simulink model "sim_quadrotor"  (R2015a)
settings: Solver=ode3  StartTime=0  StopTime=40  FixedStep=sampleTime_qcsim  MaxStep=0.1  RelTol=1e-3
InitFcn:
  | % load parameters of the default quadrotor
  | disp('Quadrotor parameters loaded by InitFcn')
  | paramsFilters %load mdl_quadcopter as well!
  | 
  | % change to Simulation folder if in data folder
  | cd([matlabpath '/Simulation']);
values from neighbouring files (symbols this model uses):
  K_lqr_toMotorcmd = lqr(A,B,Q,R)    [LQRControl.m]
undefined symbols (not defined in the file or in its folder): altEstim, controlParams, Discrete, K_poleplace, ofhandle, quad, quadEDT, sampleTime_qcsim, Time, vishandle
libraries: simulink x29, ctrlSharedLib x3, commnoisgen2 x1
(part 1 of 2)
settings Model: CovSFcnEnable=off  Creator=corkep  LastModifiedBy=root
settings DataIOCC: LimitDataPoints=off  SaveFormat=StructureWithTime  SignalLoggingSaveFormat=ModelDataLogs  SignalLogging=off  DSMLogging=off
settings OptimizationCC: ExpressionDepthLimit=2147483647  OptimizeModelRefInitCode=on  LifeSpan=1
settings DebuggingCC: UnderspecifiedInitializationDetection=Classic  MergeDetectMultiDrivingBlocksExec=none  SolverPrmCheckMsg=warning  FcnCallInpInsideContextMsg=UseLocalSettings  StateNameClashWarn=warning
settings HardwareCC: TargetBitPerLong=64  TargetBitPerPointer=64  TargetLongLongMode=on  TargetIntDivRoundTo=Zero  TargetEndianess=LittleEndian  TargetWordSize=64  TargetHWDeviceType=MATLAB Host  ProdEqTarget=off
settings RTWCC: SystemTargetFile=ert_shrlib.tlc  GenCodeOnly=on  MakeCommand="make_rtw OPTS=\"-DDEFAULT_BUFFER_SIZE=4600\""  GenerateMakefile=off  TemplateMakefile=ert_default_tmf  Description=Embedded Coder (host-based shared library target)  BuildConfiguration=Faster Runs  RTWCompilerOptimization=on
settings CodeAppCC: IgnoreCustomStorageClasses=off
settings STFCustomTargetCC: ParMdlRefBuildCompliant=on  CompOptLevelCompliant=on  IncludeMdlTerminateFcn=off  CombineOutputUpdateFcns=on  MatFileLogging=on  MultiInstanceERTCode=on  CodeInterfacePackaging=Reusable function  SupportContinuousTime=off  SupportVariableSizeSignals=off  ModelStepFunctionPrototypeControlCompliant=on  SystemTargetFile=ert_shrlib.tlc
settings ERTTargetCC: ParMdlRefBuildCompliant=on  CompOptLevelCompliant=on  IncludeMdlTerminateFcn=off  MatFileLogging=on  MultiInstanceERTCode=on  CodeInterfacePackaging=Reusable function  SupportContinuousTime=off  SupportVariableSizeSignals=off  ModelStepFunctionPrototypeControlCompliant=on  MultiInstanceErrorCode=Warning  ERTCustomFileTemplate=example_file_process.tlc

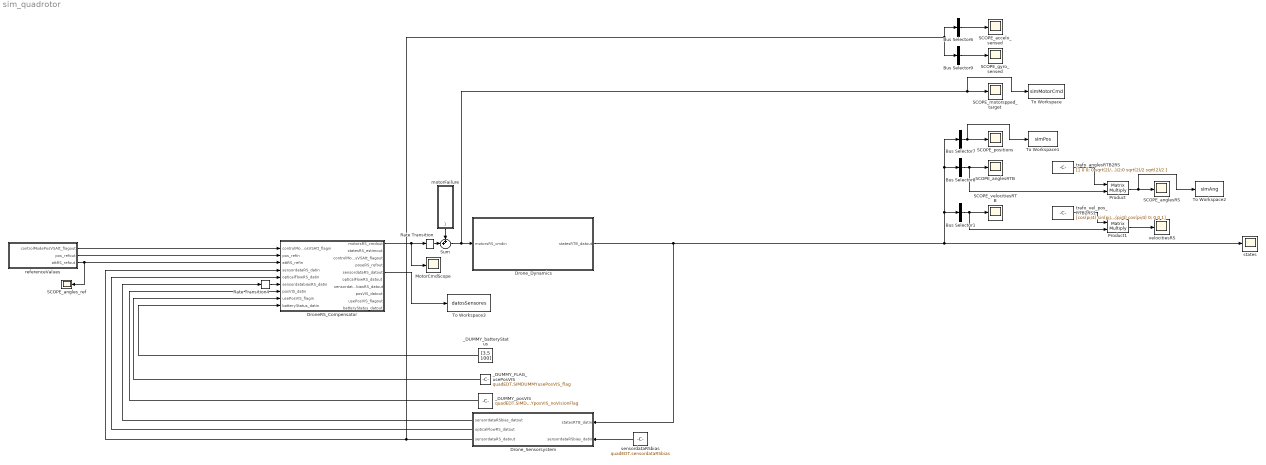
== system sim_quadrotor ==
  Bus Selector1 : BusSelector  OutputSignals=dx,dy,dz  OutputAsBus=on
  Bus Selector6 : BusSelector  OutputSignals=ddx,ddy,ddz  OutputAsBus=on
  Bus Selector7 : BusSelector  OutputSignals=X,Y,Z  OutputAsBus=on
  Bus Selector8 : BusSelector  OutputSignals=yaw,pitch,roll  OutputAsBus=on
  Bus Selector9 : BusSelector  OutputSignals=p,q,r  OutputAsBus=on
  DroneRS_Compensator : Subsystem  TreatAsAtomicUnit=on
  Drone_Dynamics : Subsystem  AncestorBlock=roblocks/Dynamics/Quadrotor
  Drone_Sensorsystem : Subsystem
  "MotorCmdScope " : Scope
      settings: YMin=-300  YMax=300  SaveName=ScopeData6
  Product : Product  Multiplication=Matrix(*)
  Product1 : Product  Multiplication=Matrix(*)
  Rate Transition : RateTransition
  Rate Transition4 : RateTransition  OutPortSampleTime=sampleTime_qcsim
  SCOPE_accelo_sensed : Scope
      settings: TimeRange=14.995  YMin=-13  YMax=2  SaveName=ScopeData11
  SCOPE_anglesRS : Scope
      settings: TimeRange=9.635  YMin=-0.09  YMax=0.06  SaveName=ScopeData8
  SCOPE_anglesRTB : Scope
      settings: TimeRange=10.425  YMin=-0.04  YMax=0.11  SaveName=ScopeData5
  SCOPE_angles_ref : Scope
      settings: TimeRange=15  YMin=-0.15  YMax=0.2  SaveName=ScopeData28
  SCOPE_gyro_sensed : Scope
      settings: TimeRange=14.995  YMin=-0.002  YMax=0.00175  SaveName=ScopeData10
  SCOPE_motorspped_target : Scope
      settings: TimeRange=9.040000000000001  YMin=-400  YMax=400  SaveName=ScopeData2
  SCOPE_positions : Scope
      settings: TimeRange=9.040000000000001  YMin=-0.8  YMax=0.3  SaveName=ScopeData3
  SCOPE_velocitiesRTB : Scope
      settings: TimeRange=13.045  YMin=-1.5  YMax=0.5  SaveName=ScopeData22
  Sum : Sum  Inputs=++|
  To Workspace : ToWorkspace  VariableName=simMotorCmd  SaveFormat=Timeseries  SampleTime=-1
  To Workspace1 : ToWorkspace  VariableName=simPos  SaveFormat=Timeseries  SampleTime=-1
  To Workspace2 : ToWorkspace  VariableName=simAng  SaveFormat=Timeseries  SampleTime=-1
  To Workspace3 : ToWorkspace  VariableName=datosSensores  SaveFormat=Timeseries  SampleTime=-1
  _DUMMY_FLAG_usePosVIS : Constant  Value=quadEDT.SIMDUMMYusePosVIS_flag
  _DUMMY_batteryStatus : Constant  Value=[3.5 100]
  _DUMMY_posVIS : Constant  Value=quadEDT.SIMDUMMYposVIS_noVisionFlag
  motorFailure : Subsystem
  referenceValues : Subsystem
  sensordataRSbias : Constant  Value=quadEDT.sensordataRSbias
  states : Scope
      settings: TimeRange=20  YMin=-1.2  YMax=0.2  SaveName=ScopeData7
  trafo_anglesRTB2RS : Constant  Value=[1 0 0; 0 sqrt(2)/2 -sqrt(2)/2;0 sqrt(2)/2 sqrt(2)/2 ]
  trafo_vel_pos_RTB2RS1 : Constant  Value=[cos(pi/4) sin(pi/4) 0 ; -sin(pi/4) cos(pi/4) 0; 0 0 1]
  velocitiesRS : Scope
      settings: TimeRange=8.18  YMin=-4.991831340204151  YMax=1.573556915322435  SaveName=ScopeData39
  wires:
  Bus Selector7/1 -> To Workspace1/1, SCOPE_positions/1
  Bus Selector8/1 -> Product/2, SCOPE_anglesRTB/1
  Bus Selector6/1 -> SCOPE_accelo_sensed/1
  Bus Selector9/1 -> SCOPE_gyro_sensed/1
  DroneRS_Compensator/1(motorsRS_cmdout) -> "MotorCmdScope "/1, Rate Transition/1
  referenceValues/2("pos_refout ") -> DroneRS_Compensator/2(pos_refin)
  Sum/1 -> To Workspace/1, SCOPE_motorspped_target/1, Drone_Dynamics/1(motorsRS_cmdin)
  motorFailure/1(motorRS_cmdout) -> Sum/1
  Rate Transition/1 -> Sum/2
  referenceValues/1(controlModePosVSAtt_flagout) -> DroneRS_Compensator/1(controlModePosVSAtt_flagin)
  referenceValues/3(attRS_refout) -> DroneRS_Compensator/3(attRS_refin), SCOPE_angles_ref/1
  Drone_Dynamics/1(statesRTB_datout) -> Drone_Sensorsystem/1(statesRTB_datin), states/1, Bus Selector1/1, Bus Selector8/1, Bus Selector7/1
  sensordataRSbias/1 -> Drone_Sensorsystem/2(sensordataRSbias_datin)
  Drone_Sensorsystem/2(opticalFlowRS_datout) -> DroneRS_Compensator/5(opticalFlowRS_datin)
  Rate Transition4/1 -> DroneRS_Compensator/6(sensordatabiasRS_datin)
  Drone_Sensorsystem/3(sensordataRS_datout) -> Bus Selector9/1, Bus Selector6/1, DroneRS_Compensator/4(sensordataRS_datin)
  Drone_Sensorsystem/1(sensordataRSbias_datout) -> Rate Transition4/1
  Product/1 -> To Workspace2/1, SCOPE_anglesRS/1
  trafo_anglesRTB2RS/1 -> Product/1
  _DUMMY_posVIS/1 -> DroneRS_Compensator/7(posVIS_datin)
  Bus Selector1/1 -> Product1/2, SCOPE_velocitiesRTB/1
  Product1/1 -> velocitiesRS/1
  _DUMMY_FLAG_usePosVIS/1 -> DroneRS_Compensator/8(usePosVIS_flagin)
  trafo_vel_pos_RTB2RS1/1 -> Product1/1
  _DUMMY_batteryStatus/1 -> DroneRS_Compensator/9(batteryStatus_datin)
  DroneRS_Compensator/5(sensordataRS_datout) -> To Workspace3/1

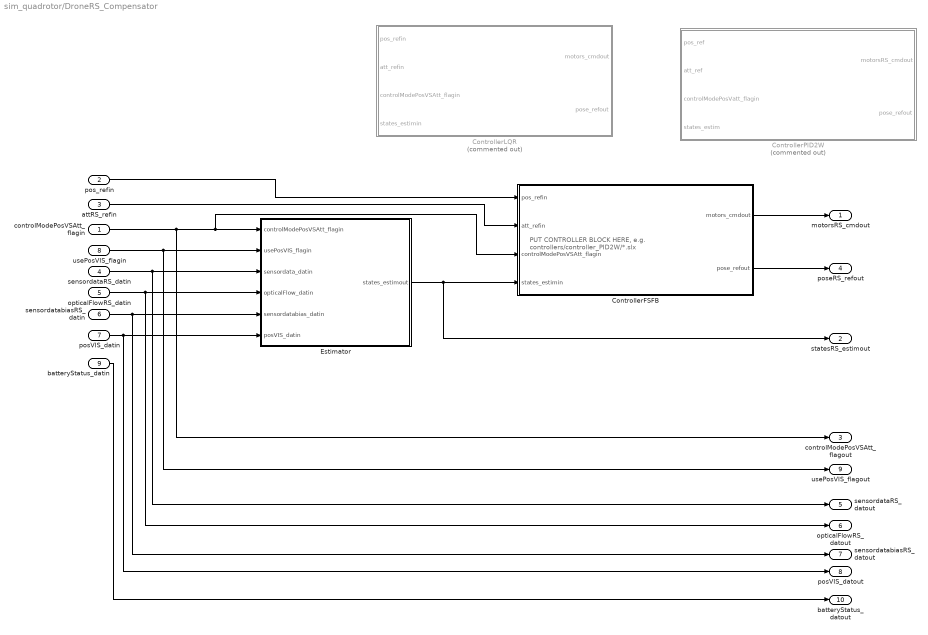
== system sim_quadrotor/DroneRS_Compensator ==
  note: PUT CONTROLLER BLOCK HERE,
      | e.g. controllers/controller_PID2W/*.slx
  controlModePosVSAtt_flagin : Inport
  pos_refin : Inport  Port=2
  attRS_refin : Inport  Port=3
  sensordataRS_datin : Inport  Port=4
  opticalFlowRS_datin : Inport  Port=5
  sensordatabiasRS_datin : Inport  Port=6
  posVIS_datin : Inport  Port=7
  usePosVIS_flagin : Inport  Port=8
  batteryStatus_datin : Inport  Port=9
  ControllerFSFB : Subsystem  TreatAsAtomicUnit=on
  ControllerLQR : Subsystem  Commented=on  TreatAsAtomicUnit=on
  ControllerPID2W : Subsystem  Commented=on  TreatAsAtomicUnit=on
  Estimator : Subsystem
  motorsRS_cmdout : Outport
  statesRS_estimout : Outport  Port=2
  controlModePosVSAtt_flagout : Outport  Port=3
  poseRS_refout : Outport  Port=4
  sensordataRS_datout : Outport  Port=5
  opticalFlowRS_datout : Outport  Port=6
  sensordatabiasRS_datout : Outport  Port=7
  posVIS_datout : Outport  Port=8
  usePosVIS_flagout : Outport  Port=9
  batteryStatus_datout : Outport  Port=10
  wires:
  sensordataRS_datin/1 -> sensordataRS_datout/1, Estimator/3(sensordata_datin)
  pos_refin/1 -> ControllerFSFB/1(pos_refin)
  Estimator/1(states_estimout) -> ControllerFSFB/4(states_estimin), statesRS_estimout/1
  attRS_refin/1 -> ControllerFSFB/2(att_refin)
  controlModePosVSAtt_flagin/1 -> controlModePosVSAtt_flagout/1, ControllerFSFB/3(controlModePosVSAtt_flagin), Estimator/1(controlModePosVSAtt_flagin)
  sensordatabiasRS_datin/1 -> Estimator/5(sensordatabias_datin), sensordatabiasRS_datout/1
  opticalFlowRS_datin/1 -> Estimator/4(opticalFlow_datin), opticalFlowRS_datout/1
  posVIS_datin/1 -> Estimator/6(posVIS_datin), posVIS_datout/1
  usePosVIS_flagin/1 -> usePosVIS_flagout/1, Estimator/2(usePosVIS_flagin)
  batteryStatus_datin/1 -> batteryStatus_datout/1
  ControllerFSFB/1(motors_cmdout) -> motorsRS_cmdout/1
  ControllerFSFB/2(pose_refout) -> poseRS_refout/1

== system sim_quadrotor/Drone_Dynamics ==
  motorsRS_cmdin : Inport
  Bus Creator : BusCreator  Inputs='X','Y','Z','yaw','pitch','roll','dx','dy','dz','p','q','r'
  Demux : Demux  Outputs=12
  Dynamics (Robotics Toolbox Peter Corke) : S-Function  FunctionName=quadrotor_dynamics  Parameters=quad
  MotorsRSToW : Subsystem
  statesRTB_datout : Outport
  wires:
  Demux/1 -> Bus Creator/1  "X"
  Demux/3 -> Bus Creator/3  "Z"
  Demux/4 -> Bus Creator/4  "yaw"
  Demux/5 -> Bus Creator/5  "pitch"
  motorsRS_cmdin/1 -> MotorsRSToW/1(motorsRS_cmdin)
  Demux/7 -> Bus Creator/7  "dx"
  Demux/9 -> Bus Creator/9  "dz"
  Demux/2 -> Bus Creator/2  "Y"
  Demux/6 -> Bus Creator/6  "roll"
  Demux/8 -> Bus Creator/8  "dy"
  Bus Creator/1 -> statesRTB_datout/1
  Dynamics (Robotics Toolbox Peter Corke)/1 -> Demux/1
  Demux/10 -> Bus Creator/10  "p"
  Demux/11 -> Bus Creator/11  "q"
  Demux/12 -> Bus Creator/12  "r"
  MotorsRSToW/1(omega_cmdout) -> Dynamics (Robotics Toolbox Peter Corke)/1

== system sim_quadrotor/Drone_Sensorsystem ==
  statesRTB_datin : Inport
  sensordataRSbias_datin : Inport  Port=2
  IMU_Pressure : Subsystem
  Rate Transition1 : RateTransition  OutPortSampleTime=sampleTime_qcsim
  Rate Transition2 : RateTransition  OutPortSampleTime=sampleTime_qcsim
  camera : Subsystem
  sensordataRSbias_datout : Outport
  opticalFlowRS_datout : Outport  Port=2
  sensordataRS_datout : Outport  Port=3
  wires:
  statesRTB_datin/1 -> IMU_Pressure/2(statesRTB_datin), camera/1(statesRTB_datin)
  sensordataRSbias_datin/1 -> sensordataRSbias_datout/1, IMU_Pressure/1(sensordataRSbias_datin)
  Rate Transition2/1 -> sensordataRS_datout/1
  Rate Transition1/1 -> opticalFlowRS_datout/1
  IMU_Pressure/1(sensordataRS_datout) -> Rate Transition2/1
  camera/1(opticalFlowRS_datout) -> Rate Transition1/1

== system sim_quadrotor/motorFailure ==
  Constant : Constant  Value=0
  Constant1 : Constant  Value=0
  Mux1 : Mux
  Step : Step  Time=quadEDT.motorFailure_time  SampleTime=0
  Step1 : Step  Time=quadEDT.motorFailure_time + quadEDT.motorFailure_duration  SampleTime=0
  Sum : Sum  Inputs=|+-
  motorFailure_gainm2 : Gain  Gain=quadEDT.motorFailure_gainm2
  motorFailure_gainm3 : Gain  Gain=quadEDT.motorFailure_gainm3
  motorRS_cmdout : Outport
  wires:
  Step/1 -> Sum/1
  Step1/1 -> Sum/2
  Sum/1 -> motorFailure_gainm3/1, motorFailure_gainm2/1
  Constant/1 -> Mux1/1
  motorFailure_gainm2/1 -> Mux1/2
  motorFailure_gainm3/1 -> Mux1/3
  Constant1/1 -> Mux1/4
  Mux1/1 -> motorRS_cmdout/1

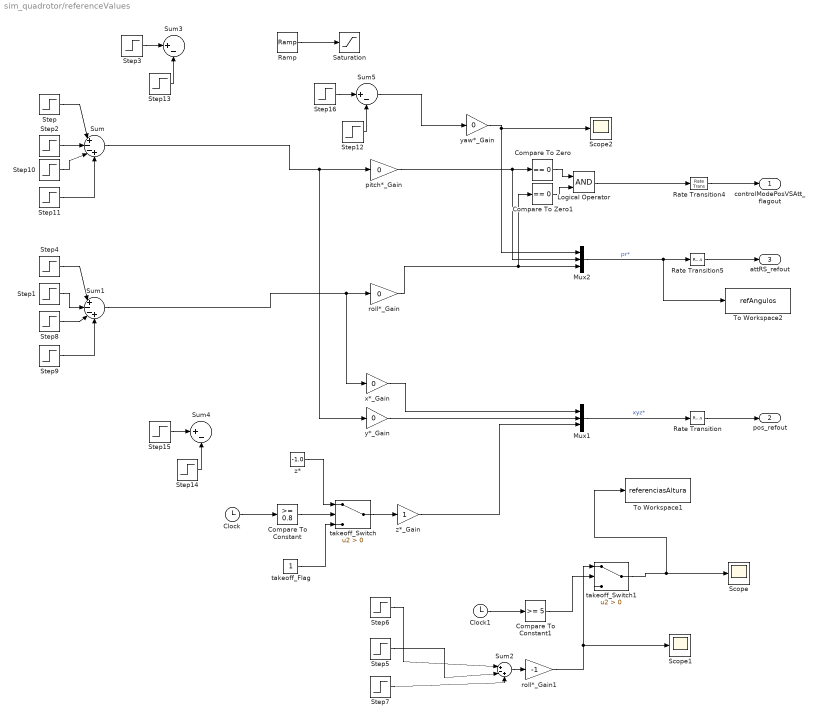
== system sim_quadrotor/referenceValues ==
  Clock : Clock
  Clock1 : Clock
  Compare To Constant : simulink/Logic and Bit Operations/Compare To Constant  relop=>=  const=0.8  OutDataTypeStr=boolean
  Compare To Constant1 : simulink/Logic and Bit Operations/Compare To Constant  relop=>=  const=5  OutDataTypeStr=boolean
  Compare To Zero : simulink/Logic and Bit Operations/Compare To Zero  relop===  OutDataTypeStr=boolean
  Compare To Zero1 : simulink/Logic and Bit Operations/Compare To Zero  relop===  OutDataTypeStr=boolean
  Logical Operator : Logic  AllPortsSameDT=off  OutDataTypeStr=boolean
  Mux1 : Mux  Inputs=3
  Mux2 : Mux  Inputs=3
  Ramp : simulink/Sources/Ramp  slope=1  start=3  X0=0
  Rate Transition : RateTransition  OutPortSampleTime=sampleTime_qcsim
  Rate Transition4 : RateTransition  OutPortSampleTime=sampleTime_qcsim
  Rate Transition5 : RateTransition  OutPortSampleTime=sampleTime_qcsim
  Saturation : Saturate  UpperLimit=5  LowerLimit=-5
  Scope : Scope
      settings: SaveName=ScopeData16
  Scope1 : Scope
      settings: SaveName=ScopeData17
  Scope2 : Scope
      settings: SaveName=ScopeData19
  Step : Step  Time=10  SampleTime=0
  Step1 : Step  Time=8  After=1.001  SampleTime=0
  Step10 : Step  Time=20  SampleTime=0
  Step11 : Step  Time=24  SampleTime=0
  Step12 : Step  Time=18  After=1.001  SampleTime=0
  Step13 : Step  Time=6  After=1.001  SampleTime=0
  Step14 : Step  Time=12  After=1.001  SampleTime=0
  Step15 : Step  Time=9  SampleTime=0
  Step16 : Step  Time=15  SampleTime=0
  Step2 : Step  Time=13  SampleTime=0
  Step3 : Step  Time=3  SampleTime=0
  Step4 : Step  Time=5  SampleTime=0
  Step5 : Step  Time=9  SampleTime=0
  Step6 : Step  Time=5  Before=1  After=1.5  SampleTime=0
  Step7 : Step  Time=12  After=0.5  SampleTime=0
  Step8 : Step  Time=15  SampleTime=0
  Step9 : Step  Time=19  SampleTime=0
  Sum : Sum  Inputs=|+--+
  Sum1 : Sum  Inputs=|+--+
  Sum2 : Sum  Inputs=|+-+
  Sum3 : Sum  Inputs=|+-
  Sum4 : Sum  Inputs=|+-
  Sum5 : Sum  Inputs=|+-
  To Workspace1 : ToWorkspace  VariableName=referenciasAltura  SaveFormat=Timeseries  SampleTime=-1
  To Workspace2 : ToWorkspace  VariableName=refAngulos  SaveFormat=Timeseries  SampleTime=-1
  pitch*_Gain : Gain  Gain=0
  roll*_Gain : Gain  Gain=0
  roll*_Gain1 : Gain  Gain=-1
  takeoff_Flag : Constant  SampleTime=0
  takeoff_Switch : Switch  Criteria=u2 > Threshold
  takeoff_Switch1 : Switch  Criteria=u2 > Threshold
  x*_Gain : Gain  Gain=0
  y*_Gain : Gain  Gain=0
  yaw*_Gain : Gain  Gain=0
  z* : Constant  Value=-1.0  SampleTime=0
  z*_Gain : Gain
  controlModePosVSAtt_flagout : Outport
  "pos_refout " : Outport  Port=2
  attRS_refout : Outport  Port=3
  wires:
  z*/1 -> takeoff_Switch/1
  y*_Gain/1 -> Mux1/2
  Mux1/1 -> Rate Transition/1  "xyz*"
  x*_Gain/1 -> Mux1/1
  Rate Transition/1 -> "pos_refout "/1
  Rate Transition4/1 -> controlModePosVSAtt_flagout/1
  Step/1 -> Sum/1
  Mux2/1 -> To Workspace2/1, Rate Transition5/1  "pr*"
  Rate Transition5/1 -> attRS_refout/1
  Step2/1 -> Sum/2
  yaw*_Gain/1 -> Scope2/1, Mux2/1
  pitch*_Gain/1 -> Mux2/2, Compare To Zero/1
  roll*_Gain/1 -> Mux2/3, Compare To Zero1/1
  Compare To Zero/1 -> Logical Operator/1
  Compare To Zero1/1 -> Logical Operator/2
  Logical Operator/1 -> Rate Transition4/1
  Clock/1 -> Compare To Constant/1
  Compare To Constant/1 -> takeoff_Switch/2
  takeoff_Flag/1 -> takeoff_Switch/3
  takeoff_Switch/1 -> z*_Gain/1
  Clock1/1 -> Compare To Constant1/1
  Compare To Constant1/1 -> takeoff_Switch1/2
  Sum2/1 -> roll*_Gain1/1
  Step6/1 -> Sum2/1
  Step5/1 -> Sum2/2
  roll*_Gain1/1 -> takeoff_Switch1/1, Scope1/1
  takeoff_Switch1/1 -> To Workspace1/1, Scope/1
  Step7/1 -> Sum2/3
  Step10/1 -> Sum/3
  Step11/1 -> Sum/4
  z*_Gain/1 -> Mux1/3
  Sum5/1 -> yaw*_Gain/1
  Step4/1 -> Sum1/1
  Step1/1 -> Sum1/2
  Step8/1 -> Sum1/3
  Step9/1 -> Sum1/4
  Ramp/1 -> Saturation/1
  Step16/1 -> Sum5/1
  Step12/1 -> Sum5/2
  Sum/1 -> y*_Gain/1, pitch*_Gain/1
  Sum1/1 -> x*_Gain/1, roll*_Gain/1
  Step3/1 -> Sum3/1
  Step13/1 -> Sum3/2
  Step15/1 -> Sum4/1
  Step14/1 -> Sum4/2

== system sim_quadrotor/DroneRS_Compensator/ControllerFSFB ==
  pos_refin : Inport
  att_refin : Inport  Port=2
  controlModePosVSAtt_flagin : Inport  Port=3
  states_estimin : Inport  Port=4
  Add : Sum  Inputs=+-
  FullstateController : Subsystem
  Selector : Selector  InputPortWidth=12  Indices=[1:6]
  SysteminputConverter : Subsystem
  statesReferences : Subsystem
  motors_cmdout : Outport
  pose_refout : Outport  Port=2
  wires:
  Selector/1 -> pose_refout/1
  statesReferences/2(states_refout) -> Add/1, Selector/1
  controlModePosVSAtt_flagin/1 -> statesReferences/3(controlModePosVSAtt_flagin)
  states_estimin/1 -> statesReferences/4(states_estimin), Add/2
  att_refin/1 -> statesReferences/2(att_refin)
  pos_refin/1 -> statesReferences/1(pos_refin)
  Add/1 -> FullstateController/1(state_error_datin)  "state error e"
  statesReferences/1(takeoffphase_flagout) -> SysteminputConverter/1(takeoffphase_flagin)
  FullstateController/1(u_totThrust_Torques_refout) -> SysteminputConverter/2(u_totThrust_Torques_refin)
  SysteminputConverter/1(motors_cmdout) -> motors_cmdout/1

== system sim_quadrotor/DroneRS_Compensator/ControllerLQR ==
  pos_refin : Inport
  att_refin : Inport  Port=2
  controlModePosVSAtt_flagin : Inport  Port=3
  states_estimin : Inport  Port=4
  Add : Sum  Inputs=+-
  FullstateController : Subsystem
  Selector : Selector  InputPortWidth=12  Indices=[1:6]
  SysteminputConverter : Subsystem
  statesReferences : Subsystem
  motors_cmdout : Outport
  pose_refout : Outport  Port=2
  wires:
  statesReferences/2(states_refout) -> Add/1, Selector/1
  controlModePosVSAtt_flagin/1 -> statesReferences/3(controlModePosVSAtt_flagin)
  states_estimin/1 -> statesReferences/4(states_estimin), Add/2
  att_refin/1 -> statesReferences/2(att_refin)
  Add/1 -> FullstateController/1(state_error_datin)  "state error e"
  statesReferences/1(takeoffphase_flagout) -> SysteminputConverter/1(takeoffphase_flagin)
  FullstateController/1(motors_cmdout) -> SysteminputConverter/2(motors_cmdin)
  pos_refin/1 -> statesReferences/1(pos_refin)
  SysteminputConverter/1(motors_cmdout) -> motors_cmdout/1
  Selector/1 -> pose_refout/1

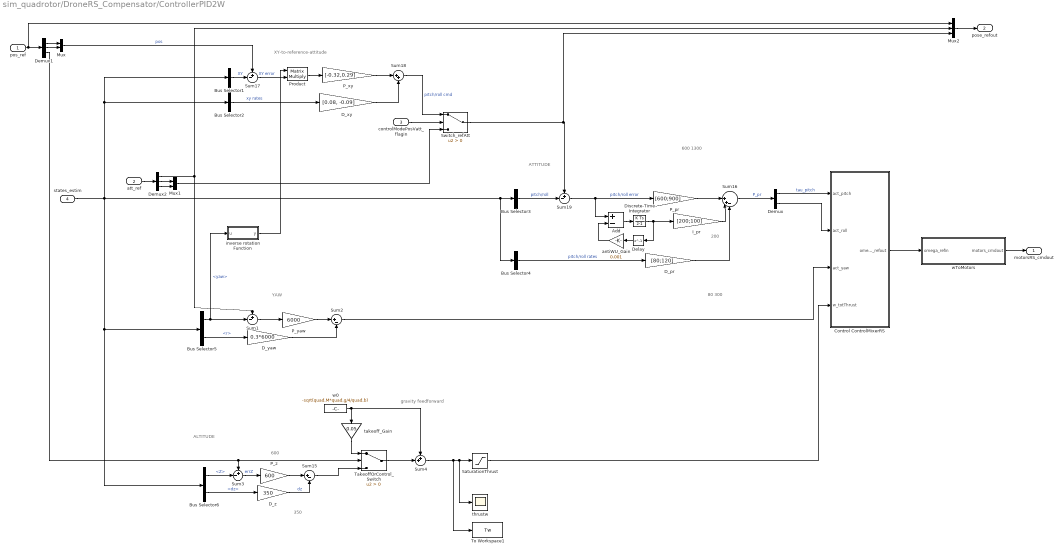
== system sim_quadrotor/DroneRS_Compensator/ControllerPID2W ==
  note: 350
  note: 600
  note: 200
  note: 80 300
  note: 600 1300
  note: XY-to-reference-attitude
  note: ALTITUDE
  note: ATTITUDE
  note: YAW
  note: gravity feedforward
  pos_ref : Inport
  att_ref : Inport  Port=2
  controlModePosVatt_flagin : Inport  Port=3
  states_estim : Inport  Port=4
  Add : Sum  Inputs=+-
  Bus Selector1 : BusSelector  OutputSignals=X,Y  OutputAsBus=on
  Bus Selector2 : BusSelector  OutputSignals=dx,dy  OutputAsBus=on
  Bus Selector3 : BusSelector  OutputSignals=pitch,roll  OutputAsBus=on
  Bus Selector4 : BusSelector  OutputSignals=q,p  OutputAsBus=on
  Bus Selector5 : BusSelector  OutputSignals=yaw,r
  Bus Selector6 : BusSelector  OutputSignals=Z,dz
  Control ControlMixerRS : Subsystem
  D_pr : Gain  Gain=[80;120]
  D_xy : Gain  Gain=[0.08, -0.09]
  D_yaw : Gain  Gain=0.3*6000
  D_z : Gain  Gain=350
  Delay : Delay  DelayLength=1  InitialCondition=0
  Demux : Demux  Outputs=2
  Demux1 : Demux  Outputs=3
  Demux2 : Demux  Outputs=3
  Discrete-Time Integrator : DiscreteIntegrator  InitialConditionSetting=State (most efficient)  SampleTime=sampleTime_qcsim  LimitOutput=on  UpperSaturationLimit=2  LowerSaturationLimit=-2
  I_pr : Gain  Gain=[200;100]
  Mux : Mux  Inputs=2
  Mux1 : Mux  Inputs=2
  Mux2 : Mux  Inputs=3
  P_pr : Gain  Gain=[600;900]
  P_xy : Gain  Gain=[-0.32,0.29]
  P_yaw : Gain  Gain=6000
  P_z : Gain  Gain=600
  Product : Product  Multiplication=Matrix(*)  RndMeth=Zero
  SaturationThrust : Saturate  UpperLimit=0.92*2618  LowerLimit=-0.92*2618
  Sum{1,3,17,19} (4 alike) : Sum  Inputs=+-|
  Sum15 : Sum  Inputs=|+-
  Sum16 : Sum  Inputs=||++-
  Sum18 : Sum  Inputs=|++
  Sum2 : Sum  Inputs=|+-
  Sum4 : Sum  Inputs=++|
  Switch_refAtt : Switch  Criteria=u2 > Threshold
  TakeoffOrControl_Switch : Switch  Criteria=u2 > Threshold
  To Workspace1 : ToWorkspace  VariableName=Tw  SampleTime=-1
  antiWU_Gain : Gain  Gain=0.001
  inverse rotation Function : MATLAB Function  TreatAsAtomicUnit=on
  takeoff_Gain : Gain  Gain=0.05
  thrustw : Scope
      settings: YMin=-0.04  YMax=0.045  SaveName=ScopeData15
  w0 : Constant  Value=-sqrt(quad.M*quad.g/4/quad.b)  SampleTime=sampleTime_qcsim
  wToMotors : Subsystem
  motorsRS_cmdout : Outport
  pose_refout : Outport  Port=2
  wires:
  w0/1 -> takeoff_Gain/1, Sum4/1
  Bus Selector2/1 -> D_xy/1  "xy rates"
  Bus Selector4/1 -> D_pr/1  "pitch/roll rates"
  Sum19/1 -> P_pr/1, Add/1  "pitch/roll error"
  Sum16/1 -> Demux/1  "P_pr"
  Bus Selector5/1 -> inverse rotation Function/1(u), Sum1/2  "<yaw>"
  Bus Selector6/1 -> Sum3/2  "<Z>"
  inverse rotation Function/1(y) -> Product/1
  Bus Selector5/2 -> D_yaw/1  "<r>"
  Sum3/1 -> P_z/1  "errZ"
  Bus Selector6/2 -> D_z/1  "<dz>"
  D_z/1 -> Sum15/2  "dz"
  D_yaw/1 -> Sum2/2
  Sum4/1 -> To Workspace1/1, thrustw/1, SaturationThrust/1
  Sum1/1 -> P_yaw/1
  Sum17/1 -> Product/2  "XY error"
  Discrete-Time Integrator/1 -> Delay/1, I_pr/1
  Demux/1 -> Control ControlMixerRS/1(act_pitch)  "tau_pitch"
  Sum2/1 -> Control ControlMixerRS/3(act_yaw)
  Demux/2 -> Control ControlMixerRS/2(act_roll)
  TakeoffOrControl_Switch/1 -> Sum4/2
  Sum15/1 -> TakeoffOrControl_Switch/3
  takeoff_Gain/1 -> TakeoffOrControl_Switch/1
  Sum18/1 -> Switch_refAtt/1  "pitch/roll cmd"
  controlModePosVatt_flagin/1 -> Switch_refAtt/2
  pos_ref/1 -> Mux2/1, Demux1/1
  Demux1/1 -> Mux/1
  Demux1/2 -> Mux/2
  Mux/1 -> Sum17/1  "pos"
  Demux2/2 -> Mux1/1
  Demux2/3 -> Mux1/2
  att_ref/1 -> Demux2/1
  Mux1/1 -> Switch_refAtt/3
  Demux2/1 -> Mux2/2, Sum1/1
  Demux1/3 -> Sum3/1, TakeoffOrControl_Switch/2
  Bus Selector3/1 -> Sum19/2  "pitch/roll"
  Product/1 -> P_xy/1
  D_xy/1 -> Sum18/2
  Bus Selector1/1 -> Sum17/2  "XY"
  P_z/1 -> Sum15/1
  SaturationThrust/1 -> Control ControlMixerRS/4(w_totThrust)
  P_yaw/1 -> Sum2/1
  I_pr/1 -> Sum16/2
  D_pr/1 -> Sum16/3
  P_pr/1 -> Sum16/1
  Control ControlMixerRS/1(omega_refout) -> wToMotors/1(omega_refin)
  wToMotors/1(motors_cmdout) -> motorsRS_cmdout/1
  Mux2/1 -> pose_refout/1
  Switch_refAtt/1 -> Mux2/3, Sum19/1
  states_estim/1 -> Bus Selector4/1, Bus Selector3/1, Bus Selector1/1, Bus Selector2/1, Bus Selector5/1, Bus Selector6/1
  P_xy/1 -> Sum18/1
  Add/1 -> Discrete-Time Integrator/1
  antiWU_Gain/1 -> Add/2
  Delay/1 -> antiWU_Gain/1

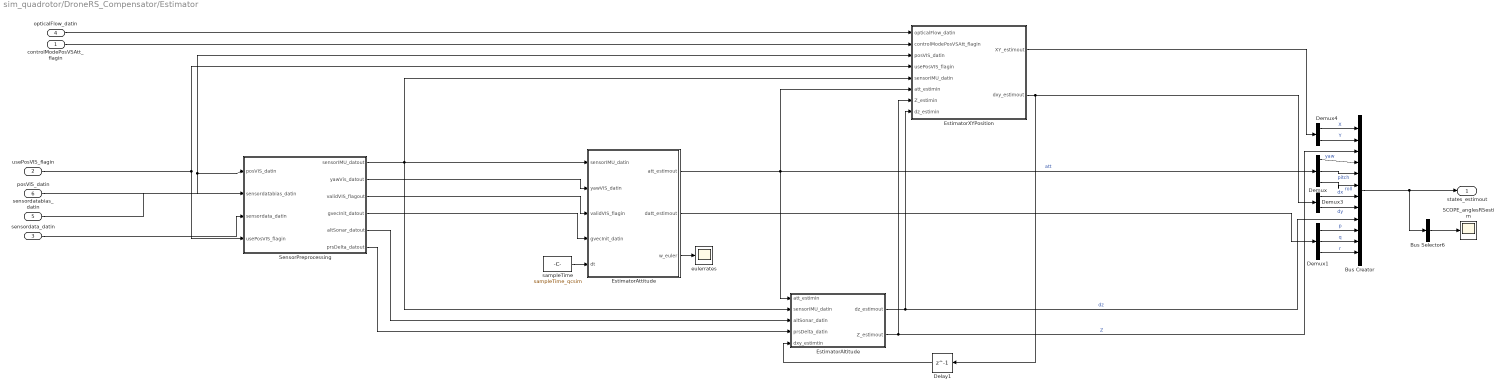
== system sim_quadrotor/DroneRS_Compensator/Estimator ==
  controlModePosVSAtt_flagin : Inport
  usePosVIS_flagin : Inport  Port=2
  sensordata_datin : Inport  Port=3
  opticalFlow_datin : Inport  Port=4
  sensordatabias_datin : Inport  Port=5
  posVIS_datin : Inport  Port=6
  Bus Creator : BusCreator  Inputs='X','Y','Z','yaw','pitch','roll','dx','dy','dz','p','q','r'
  Bus Selector6 : BusSelector  OutputSignals=yaw,pitch,roll  OutputAsBus=on
  Delay1 : Delay  DelayLength=1  InitialCondition=0
  Demux : Demux  Outputs=3
  Demux1 : Demux  Outputs=3
  Demux3 : Demux  Outputs=2
  Demux4 : Demux  Outputs=2
  EstimatorAltitude : Subsystem
  EstimatorAttitude : MATLAB Function  TreatAsAtomicUnit=on
  EstimatorXYPosition : Subsystem
  SCOPE_anglesRSestim : Scope
      settings: TimeRange=3.57  YMin=-0.08  YMax=0.06000000000000001  SaveName=ScopeData4
  SensorPreprocessing : Subsystem
  eulerrates : Scope
      settings: SaveName=ScopeData18
  sampleTime : Constant  Value=sampleTime_qcsim
  states_estimout : Outport
  wires:
  Bus Creator/1 -> Bus Selector6/1, states_estimout/1
  sampleTime/1 -> EstimatorAttitude/5(dt)
  sensordatabias_datin/1 -> SensorPreprocessing/2(sensordatabias_datin)
  EstimatorAttitude/3(w_euler) -> eulerrates/1
  EstimatorAltitude/2(Z_estimout) -> Bus Creator/3, EstimatorXYPosition/7(Z_estimin)  "Z"
  EstimatorAltitude/1(dz_estimout) -> Bus Creator/9, EstimatorXYPosition/8(dz_estimin)  "dz"
  opticalFlow_datin/1 -> EstimatorXYPosition/1(opticalFlow_datin)
  Demux3/1 -> Bus Creator/7  "dx"
  Demux3/2 -> Bus Creator/8  "dy"
  EstimatorXYPosition/2(dxy_estimout) -> Delay1/1, Demux3/1
  Delay1/1 -> EstimatorAltitude/5(dxy_estimtin)
  controlModePosVSAtt_flagin/1 -> EstimatorXYPosition/2(controlModePosVSAtt_flagin)
  Demux4/1 -> Bus Creator/1  "X"
  Demux4/2 -> Bus Creator/2  "Y"
  EstimatorXYPosition/1(XY_estimout) -> Demux4/1
  posVIS_datin/1 -> EstimatorXYPosition/3(posVIS_datin), SensorPreprocessing/1(posVIS_datin)
  usePosVIS_flagin/1 -> SensorPreprocessing/4(usePosVIS_flagin), EstimatorXYPosition/4(usePosVIS_flagin)
  Bus Selector6/1 -> SCOPE_anglesRSestim/1
  SensorPreprocessing/1(sensorIMU_datout) -> EstimatorAltitude/2(sensorIMU_datin), EstimatorXYPosition/5(sensorIMU_datin), EstimatorAttitude/1(sensorIMU_datin)
  SensorPreprocessing/4(gvecInit_datout) -> EstimatorAttitude/4(gvecInit_datin)
  sensordata_datin/1 -> SensorPreprocessing/3(sensordata_datin)
  SensorPreprocessing/5(altSonar_datout) -> EstimatorAltitude/3(altSonar_datin)
  SensorPreprocessing/6(prsDelta_datout) -> EstimatorAltitude/4(prsDelta_datin)
  EstimatorAttitude/1(att_estimout) -> EstimatorAltitude/1(att_estimin), Demux/1, EstimatorXYPosition/6(att_estimin)  "att"
  Demux/1 -> Bus Creator/4  "yaw"
  Demux/2 -> Bus Creator/5  "pitch"
  Demux/3 -> Bus Creator/6  "roll"
  Demux1/1 -> Bus Creator/10  "p"
  Demux1/2 -> Bus Creator/11  "q"
  Demux1/3 -> Bus Creator/12  "r"
  EstimatorAttitude/2(datt_estimout) -> Demux1/1
  SensorPreprocessing/3(validVIS_flagout) -> EstimatorAttitude/3(validVIS_flagin)
  SensorPreprocessing/2(yawVis_datout) -> EstimatorAttitude/2(yawVIS_datin)

== system sim_quadrotor/Drone_Dynamics/MotorsRSToW ==
  motorsRS_cmdin : Inport
  Signed Sqrt : Sqrt  Operator=signedSqrt  SaturateOnIntegerOverflow=on
  motorsRSToW2_Gain : Gain  Gain=quadEDT.motorsRSToW2_Gain
  omega_cmdout : Outport
  wires:
  motorsRSToW2_Gain/1 -> Signed Sqrt/1
  motorsRS_cmdin/1 -> motorsRSToW2_Gain/1
  Signed Sqrt/1 -> omega_cmdout/1

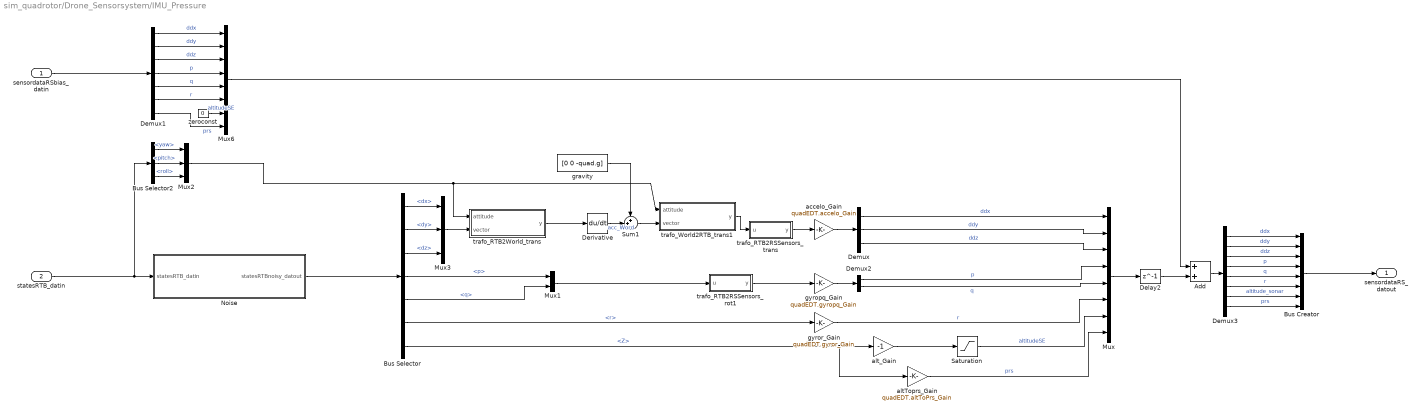
== system sim_quadrotor/Drone_Sensorsystem/IMU_Pressure ==
  sensordataRSbias_datin : Inport
  statesRTB_datin : Inport  Port=2
  " Noise" : Subsystem
  Add : Sum
  Bus Creator : BusCreator  Inputs=8
  Bus Selector : BusSelector  OutputSignals=dx,dy,dz,p,q,r,Z
  Bus Selector2 : BusSelector  OutputSignals=yaw,pitch,roll
  Delay2 : Delay  DelayLength=1  InitialCondition=0
  Demux : Demux  Outputs=3
  Demux1 : Demux  Outputs=7
  Demux2 : Demux  Outputs=2
  Demux3 : Demux  Outputs=8
  Derivative : Derivative
  Mux : Mux  Inputs=8
  Mux1 : Mux  Inputs=2
  Mux2 : Mux  Inputs=3
  Mux3 : Mux  Inputs=3
  Mux6 : Mux  Inputs=8
  Saturation : Saturate  UpperLimit=inf  LowerLimit=quadEDT.altSenor_LowerLimit
  Sum1 : Sum  Inputs=++|
  accelo_Gain : Gain  Gain=quadEDT.accelo_Gain
  altToprs_Gain : Gain  Gain=quadEDT.altToPrs_Gain
  alt_Gain : Gain  Gain=-1
  gravity : Constant  Value=[0 0 -quad.g]
  gyropq_Gain : Gain  Gain=quadEDT.gyropq_Gain
  gyror_Gain : Gain  Gain=quadEDT.gyror_Gain
  trafo_RTB2RSSensors_rot1 : MATLAB Function  TreatAsAtomicUnit=on
  trafo_RTB2RSSensors_trans : MATLAB Function  TreatAsAtomicUnit=on
  trafo_RTB2World_trans : MATLAB Function  TreatAsAtomicUnit=on
  trafo_World2RTB_trans1 : MATLAB Function  TreatAsAtomicUnit=on
  zeroconst : Constant  Value=0
  sensordataRS_datout : Outport
  wires:
  statesRTB_datin/1 -> " Noise"/1(statesRTB_datin), Bus Selector2/1
  sensordataRSbias_datin/1 -> Demux1/1
  Demux2/2 -> Mux/5  "q"
  Demux2/1 -> Mux/4  "p"
  " Noise"/1(statesRTBnoisy_datout) -> Bus Selector/1
  Bus Selector/2 -> Mux3/2  "<dy>"
  trafo_RTB2RSSensors_trans/1(y) -> accelo_Gain/1
  Demux/1 -> Mux/1  "ddx"
  Demux/2 -> Mux/2  "ddy"
  gyror_Gain/1 -> Mux/6  "r"
  Bus Selector2/1 -> Mux2/1  "<yaw>"
  Bus Selector2/2 -> Mux2/2  "<pitch>"
  Bus Selector2/3 -> Mux2/3  "<roll>"
  Demux/3 -> Mux/3  "ddz"
  Mux2/1 -> trafo_World2RTB_trans1/1(attitude), trafo_RTB2World_trans/1(attitude)
  gravity/1 -> Sum1/1
  Mux1/1 -> trafo_RTB2RSSensors_rot1/1(u)
  Bus Selector/4 -> Mux1/1  "<p>"
  Bus Selector/5 -> Mux1/2  "<q>"
  Bus Selector/6 -> gyror_Gain/1  "<r>"
  Bus Selector/7 -> altToprs_Gain/1, alt_Gain/1  "<Z>"
  alt_Gain/1 -> Saturation/1
  Saturation/1 -> Mux/7  "altitudeSE"
  Bus Selector/3 -> Mux3/3  "<dz>"
  altToprs_Gain/1 -> Mux/8  "prs"
  Demux1/1 -> Mux6/1  "ddx"
  Demux1/2 -> Mux6/2  "ddy"
  Demux1/3 -> Mux6/3  "ddz"
  Demux1/4 -> Mux6/4  "p"
  Demux1/5 -> Mux6/5  "q"
  Demux1/6 -> Mux6/6  "r"
  zeroconst/1 -> Mux6/7  "altitudeSE"
  Demux1/7 -> Mux6/8  "prs"
  Mux6/1 -> Add/1
  Add/1 -> Demux3/1
  Mux/1 -> Delay2/1
  Demux3/3 -> Bus Creator/3  "ddz"
  Demux3/1 -> Bus Creator/1  "ddx"
  Demux3/2 -> Bus Creator/2  "ddy"
  Demux3/4 -> Bus Creator/4  "p"
  Demux3/5 -> Bus Creator/5  "q"
  Demux3/6 -> Bus Creator/6  "r"
  Demux3/7 -> Bus Creator/7  "altitude_sonar"
  Demux3/8 -> Bus Creator/8  "prs"
  Bus Creator/1 -> sensordataRS_datout/1
  trafo_RTB2RSSensors_rot1/1(y) -> gyropq_Gain/1
  Bus Selector/1 -> Mux3/1  "<dx>"
  Delay2/1 -> Add/2
  accelo_Gain/1 -> Demux/1
  gyropq_Gain/1 -> Demux2/1
  Mux3/1 -> trafo_RTB2World_trans/2(vector)
  trafo_RTB2World_trans/1(y) -> Derivative/1
  Sum1/1 -> trafo_World2RTB_trans1/2(vector)
  Derivative/1 -> Sum1/2  "acc_Word"
  trafo_World2RTB_trans1/1(y) -> trafo_RTB2RSSensors_trans/1(u)

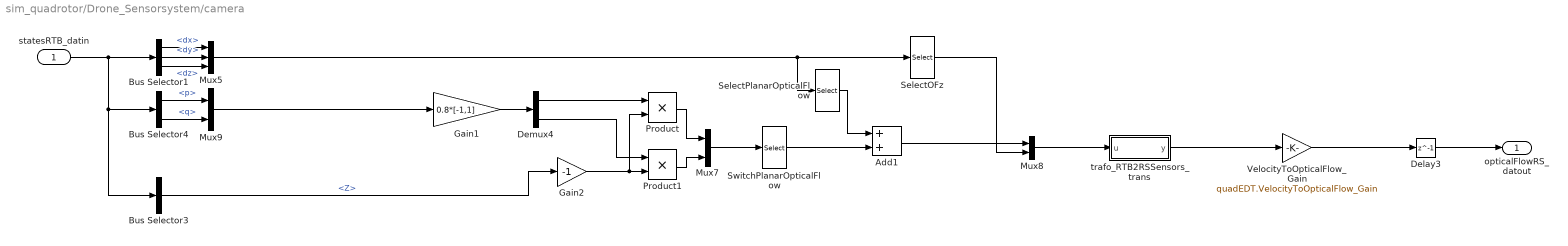
== system sim_quadrotor/Drone_Sensorsystem/camera ==
  statesRTB_datin : Inport
  Add1 : Sum
  Bus Selector1 : BusSelector  OutputSignals=dx,dy,dz
  Bus Selector3 : BusSelector  OutputSignals=Z
  Bus Selector4 : BusSelector  OutputSignals=p,q
  Delay3 : Delay  DelayLength=1  InitialCondition=0
  Demux4 : Demux  Outputs=2
  Gain1 : Gain  Gain=0.8*[-1,1]
  Gain2 : Gain  Gain=-1
  Mux5 : Mux  Inputs=3
  Mux7 : Mux  Inputs=2
  Mux8 : Mux  Inputs=2
  Mux9 : Mux  Inputs=2
  Product : Product
  Product1 : Product
  SelectOFz : Selector  InputPortWidth=3  Indices=3
  SelectPlanarOpticalFlow : Selector  InputPortWidth=3  Indices=[1 2]
  SwitchPlanarOpticalFlow : Selector  InputPortWidth=2  Indices=[2 1]
  VelocityToOpticalFlow_Gain : Gain  Gain=quadEDT.VelocityToOpticalFlow_Gain
  trafo_RTB2RSSensors_trans : MATLAB Function  TreatAsAtomicUnit=on
  opticalFlowRS_datout : Outport
  wires:
  statesRTB_datin/1 -> Bus Selector3/1, Bus Selector4/1, Bus Selector1/1
  Bus Selector1/1 -> Mux5/1  "<dx>"
  Bus Selector1/2 -> Mux5/2  "<dy>"
  Bus Selector1/3 -> Mux5/3  "<dz>"
  VelocityToOpticalFlow_Gain/1 -> Delay3/1
  Mux5/1 -> SelectPlanarOpticalFlow/1, SelectOFz/1
  Demux4/1 -> Product/1
  Gain1/1 -> Demux4/1
  Demux4/2 -> Product1/1
  Product/1 -> Mux7/1
  Product1/1 -> Mux7/2
  Mux7/1 -> SwitchPlanarOpticalFlow/1
  Mux9/1 -> Gain1/1
  Gain2/1 -> Product/2, Product1/2
  SelectPlanarOpticalFlow/1 -> Add1/1
  SwitchPlanarOpticalFlow/1 -> Add1/2
  Add1/1 -> Mux8/1
  SelectOFz/1 -> Mux8/2
  Mux8/1 -> trafo_RTB2RSSensors_trans/1(u)
  Bus Selector3/1 -> Gain2/1  "<Z>"
  Bus Selector4/1 -> Mux9/1  "<p>"
  Bus Selector4/2 -> Mux9/2  "<q>"
  trafo_RTB2RSSensors_trans/1(y) -> VelocityToOpticalFlow_Gain/1
  Delay3/1 -> opticalFlowRS_datout/1

== system sim_quadrotor/DroneRS_Compensator/ControllerFSFB/FullstateController ==
  note: IMPLEMENT FULLSTATE-
      | CONTROLLER HERE
  state_error_datin : Inport
  Gain : Gain  Gain=K_poleplace  Multiplication=Matrix(K*u)
  u_totThrust_Torques_refout : Outport
  wires:
  state_error_datin/1 -> Gain/1
  Gain/1 -> u_totThrust_Torques_refout/1

== system sim_quadrotor/DroneRS_Compensator/ControllerFSFB/SysteminputConverter ==
  note: NOTE: The Systeminputconverter takes care of two things:
      | 1) During take off, adjust the total thrust proposed by the controller
      | 2) Translate the "mechanical" system inputs (total thrust, torques around body-frame x-y-z-axes) to actual motor commands.
      | This R4->R4 mapping is a simple bijective function and does not have any dynamics. This allows us to design the controller with more intuitive "mechanical inputs" (total thrust, torques) and later simple map these to actual motor commands.
  takeoffphase_flagin : Inport
  u_totThrust_Torques_refin : Inport  Port=2
  ControlMixerRS : Subsystem
  Demux3 : Demux
  Takeoffphase_Thrustadjustment : Subsystem
  Thrust2Motorcmd : Subsystem
  motors_cmdout : Outport
  wires:
  takeoffphase_flagin/1 -> Takeoffphase_Thrustadjustment/1(takeoffphase_flagin)
  Takeoffphase_Thrustadjustment/1(totThrust_refout) -> ControlMixerRS/1(T_refin)
  Demux3/1 -> Takeoffphase_Thrustadjustment/2(totThrustbyController_refin)
  u_totThrust_Torques_refin/1 -> Demux3/1
  Demux3/4 -> ControlMixerRS/4(Qroll_refin)
  Demux3/3 -> ControlMixerRS/3(Qpitch_refin)
  Demux3/2 -> ControlMixerRS/2(Qyaw_refin)
  ControlMixerRS/1(thrust_refout) -> Thrust2Motorcmd/1(thrust_refin)
  Thrust2Motorcmd/1(motors_cmdout) -> motors_cmdout/1

== system sim_quadrotor/DroneRS_Compensator/ControllerFSFB/statesReferences ==
  note: attitude-only control reference
  note: Full-pose-reference
  note: NOTE: When we want the drone to reach and maintain a given non-zero attitude,
      | we obviously do not care about errors in x-y-position . A fullstate-feedback controller, however, acts
      | on the full state-error. To avoid influences of a x-y-position error (because in attitude-only-control we don't care about it),
      | we set the x-y-reference-position to the current postition estimate (so we get a zero "x-y-position" error).
  pos_refin : Inport
  att_refin : Inport  Port=2
  controlModePosVSAtt_flagin : Inport  Port=3
  states_estimin : Inport  Port=4
  Bus Selector : BusSelector  OutputSignals=X,Y
  Bus Selector1 : BusSelector  OutputSignals=dx,dy
  Compare To Zero : simulink/Logic and Bit Operations/Compare To Zero  relop=>  OutDataTypeStr=boolean
  Mux1 : Mux  Inputs=3
  Mux3 : Mux
  Mux4 : Mux
  Mux5 : Mux  Inputs=3
  PosVSAtt_Switch : Switch  Criteria=u2 > Threshold
  Selector : Selector  InputPortWidth=3  Indices=[3]
  dz_ref : Constant  Value=0
  velocitiesPos_ref : Constant  Value=[0;0;0]
  velocitiesRot_ref : Constant  Value=[0;0;0]
  takeoffphase_flagout : Outport
  states_refout : Outport  Port=2
  wires:
  dz_ref/1 -> Mux1/3
  Mux1/1 -> Mux4/3
  Bus Selector1/2 -> Mux1/2  "<dy>"
  Bus Selector1/1 -> Mux1/1  "<dx>"
  Mux5/1 -> Mux4/1
  Mux4/1 -> PosVSAtt_Switch/3
  Bus Selector/2 -> Mux5/2  "<Y>"
  Bus Selector/1 -> Mux5/1  "<X>"
  Mux3/1 -> PosVSAtt_Switch/1
  controlModePosVSAtt_flagin/1 -> PosVSAtt_Switch/2
  Selector/1 -> Compare To Zero/1, Mux5/3
  PosVSAtt_Switch/1 -> states_refout/1
  velocitiesRot_ref/1 -> Mux4/4, Mux3/4
  velocitiesPos_ref/1 -> Mux3/3
  states_estimin/1 -> Bus Selector/1, Bus Selector1/1
  att_refin/1 -> Mux4/2, Mux3/2
  pos_refin/1 -> Mux3/1, Selector/1
  Compare To Zero/1 -> takeoffphase_flagout/1

== system sim_quadrotor/DroneRS_Compensator/ControllerLQR/FullstateController ==
  note: IMPLEMENT FULLSTATE-
      | CONTROLLER HERE
  state_error_datin : Inport
  Gain : Gain  Gain=K_lqr_toMotorcmd  Multiplication=Matrix(K*u)
  motors_cmdout : Outport
  wires:
  state_error_datin/1 -> Gain/1
  Gain/1 -> motors_cmdout/1

== system sim_quadrotor/DroneRS_Compensator/ControllerLQR/SysteminputConverter ==
  note: NOTE: The Systeminputconverter takes care of two things:
      | 1) During take off, adjust the total thrust proposed by the controller
      | 2) Translate the "mechanical" system inputs (total thrust, torques around body-frame x-y-z-axes) to actual motor commands.
      | This R4->R4 mapping is a simple bijective function and does not have any dynamics. This allows us to design the controller with more intuitive "mechanical inputs" (total thrust, torques) and later simple map these to actual motor commands.
  takeoffphase_flagin : Inport
  motors_cmdin : Inport  Port=2
  ControlMixerRS : Subsystem
  Conversion Motorcommands To TotalThrust and Torques : Subsystem
  Demux3 : Demux
  Takeoffphase_Thrustadjustment : Subsystem
  Thrust2Motorcmd : Subsystem
  motors_cmdout : Outport
  wires:
  takeoffphase_flagin/1 -> Takeoffphase_Thrustadjustment/1(takeoffphase_flagin)
  Takeoffphase_Thrustadjustment/1(totThrust_refout) -> ControlMixerRS/1(T_refin)
  Demux3/1 -> Takeoffphase_Thrustadjustment/2(totThrustbyController_refin)
  Demux3/4 -> ControlMixerRS/4(Qroll_refin)
  Demux3/3 -> ControlMixerRS/3(Qpitch_refin)
  Demux3/2 -> ControlMixerRS/2(Qyaw_refin)
  ControlMixerRS/1(thrust_refout) -> Thrust2Motorcmd/1(thrust_refin)
  Thrust2Motorcmd/1(motors_cmdout) -> motors_cmdout/1
  motors_cmdin/1 -> Conversion Motorcommands To TotalThrust and Torques/1(motors_cmdin)
  Conversion Motorcommands To TotalThrust and Torques/1(u_tthrust_torques) -> Demux3/1

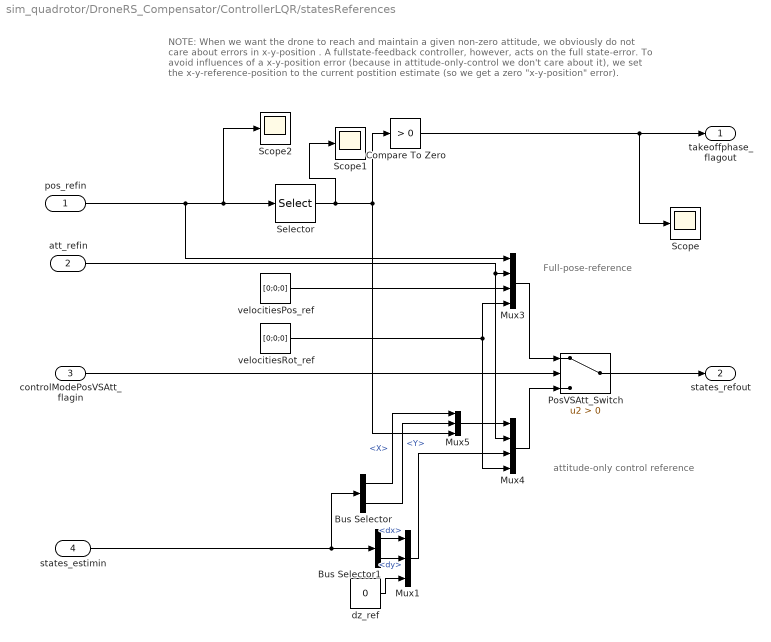
== system sim_quadrotor/DroneRS_Compensator/ControllerLQR/statesReferences ==
  note: attitude-only control reference
  note: Full-pose-reference
  note: NOTE: When we want the drone to reach and maintain a given non-zero attitude,
      | we obviously do not care about errors in x-y-position . A fullstate-feedback controller, however, acts
      | on the full state-error. To avoid influences of a x-y-position error (because in attitude-only-control we don't care about it),
      | we set the x-y-reference-position to the current postition estimate (so we get a zero "x-y-position" error).
  pos_refin : Inport
  att_refin : Inport  Port=2
  controlModePosVSAtt_flagin : Inport  Port=3
  states_estimin : Inport  Port=4
  Bus Selector : BusSelector  OutputSignals=X,Y
  Bus Selector1 : BusSelector  OutputSignals=dx,dy
  Compare To Zero : simulink/Logic and Bit Operations/Compare To Zero  relop=>  OutDataTypeStr=boolean
  Mux1 : Mux  Inputs=3
  Mux3 : Mux
  Mux4 : Mux
  Mux5 : Mux  Inputs=3
  PosVSAtt_Switch : Switch  Criteria=u2 > Threshold
  Scope : Scope
      settings: SaveName=ScopeData12
  Scope1 : Scope
      settings: SaveName=ScopeData13
  Scope2 : Scope
      settings: SaveName=ScopeData14
  Selector : Selector  InputPortWidth=3  Indices=[3]
  dz_ref : Constant  Value=0
  velocitiesPos_ref : Constant  Value=[0;0;0]
  velocitiesRot_ref : Constant  Value=[0;0;0]
  takeoffphase_flagout : Outport
  states_refout : Outport  Port=2
  wires:
  dz_ref/1 -> Mux1/3
  Mux1/1 -> Mux4/3
  Bus Selector1/2 -> Mux1/2  "<dy>"
  Bus Selector1/1 -> Mux1/1  "<dx>"
  Mux5/1 -> Mux4/1
  Mux4/1 -> PosVSAtt_Switch/3
  Bus Selector/2 -> Mux5/2  "<Y>"
  Bus Selector/1 -> Mux5/1  "<X>"
  Mux3/1 -> PosVSAtt_Switch/1
  controlModePosVSAtt_flagin/1 -> PosVSAtt_Switch/2
  Selector/1 -> Scope1/1, Compare To Zero/1, Mux5/3
  PosVSAtt_Switch/1 -> states_refout/1
  velocitiesRot_ref/1 -> Mux4/4, Mux3/4
  velocitiesPos_ref/1 -> Mux3/3
  states_estimin/1 -> Bus Selector/1, Bus Selector1/1
  att_refin/1 -> Mux4/2, Mux3/2
  pos_refin/1 -> Mux3/1, Scope2/1, Selector/1
  Compare To Zero/1 -> Scope/1, takeoffphase_flagout/1

== system sim_quadrotor/DroneRS_Compensator/ControllerPID2W/Control ControlMixerRS ==
  act_pitch : Inport
  act_roll : Inport  Port=2
  act_yaw : Inport  Port=3
  w_totThrust : Inport  Port=4
  Action2omega : Constant  Value="[0.7071, 0.7071, -1.0000, -1.00;   -0.7071,    0.7071,   -1.0000,    1.00;   -0.7071,   -0.7071,   -1.0000,   -1.00;    0.7071,   -0.7071,   -1.0000,    1.00]"
  Demux : Demux
  Gain{3..6} (4 alike) : Gain  Gain=-1
  Mux1 : Mux
  Mux2 : Mux
  Product : Product  Multiplication=Matrix(*)  RndMeth=Zero
  Saturation{1..4} (4 alike) : Saturate  UpperLimit=2618  LowerLimit=500
  omega_refout : Outport
  wires:
  Saturation3/1 -> Mux1/3
  Saturation4/1 -> Gain6/1
  Saturation2/1 -> Mux1/1
  Mux1/1 -> omega_refout/1
  Gain3/1 -> Saturation1/1
  Saturation1/1 -> Gain4/1
  Gain4/1 -> Mux1/2
  Gain5/1 -> Saturation4/1
  Gain6/1 -> Mux1/4
  act_pitch/1 -> Mux2/1
  act_roll/1 -> Mux2/2
  act_yaw/1 -> Mux2/3
  w_totThrust/1 -> Mux2/4
  Mux2/1 -> Product/2
  Action2omega/1 -> Product/1
  Product/1 -> Demux/1
  Demux/1 -> Saturation2/1
  Demux/2 -> Gain3/1
  Demux/3 -> Saturation3/1
  Demux/4 -> Gain5/1

== system sim_quadrotor/DroneRS_Compensator/ControllerPID2W/wToMotors ==
  omega_refin : Inport
  Math Function : Math  Operator=square  SaturateOnIntegerOverflow=on
  Product1 : Product
  Sign : Signum
  w2MotorsQF_Gain : Gain  Gain=0.0085
  motors_cmdout : Outport
  wires:
  omega_refin/1 -> w2MotorsQF_Gain/1
  Math Function/1 -> Product1/1
  Product1/1 -> motors_cmdout/1
  w2MotorsQF_Gain/1 -> Sign/1, Math Function/1
  Sign/1 -> Product1/2

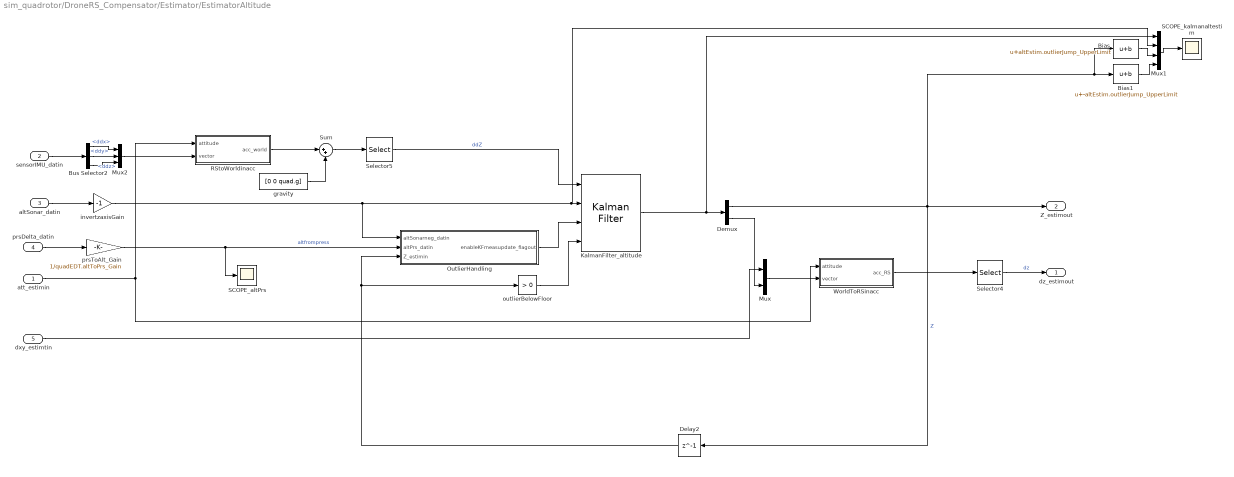
== system sim_quadrotor/DroneRS_Compensator/Estimator/EstimatorAltitude ==
  att_estimin : Inport
  sensorIMU_datin : Inport  Port=2
  altSonar_datin : Inport  Port=3
  prsDelta_datin : Inport  Port=4
  dxy_estimtin : Inport  Port=5
  Bias : Bias  Bias=altEstim.outlierJump_UpperLimit
  Bias1 : Bias  Bias=-altEstim.outlierJump_UpperLimit
  Bus Selector2 : BusSelector  OutputSignals=ddx,ddy,ddz
  Delay2 : Delay  DelayLength=1  InitialCondition=0
  Demux : Demux  Outputs=2
  KalmanFilter_altitude : ctrlSharedLib/Kalman Filter  TimeDomain=Discrete-Time  UseCurrentEstimator=on  ModelSource=Individual A, B, C, D matrices  ModelSourceVariable=sys  A=[1 sampleTime_qcsim; 0 1]  B=[0;sampleTime_qcsim]  C=[1 0]  D=[0]  NumberOfStates=2  NumberOfInputs=2  NumberOfOutputs=2  InitialEstimateSource=Dialog  X0=[-0.046 0]  P0=10  UseK=off  UseGH=on  NumberOfProcessNoiseInputs=2  G=[0;1]  TimeInvariantG=on  H=0  TimeInvariantH=on  Q=0.0005  TimeInvariantQ=on  R=[0.1]  TimeInvariantR=on  N=0  TimeInvariantN=on  AddInputPort=on  AddEnablePort=on  ExternalReset=Level hold  OutputEstimatedY=off  OutputP=off  Ts=-1
  Mux : Mux  Inputs=2
  Mux1 : Mux
  Mux2 : Mux  Inputs=3
  OutlierHandling : Subsystem
  RStoWorldinacc : MATLAB Function  TreatAsAtomicUnit=on
  SCOPE_altPrs : Scope
      settings: TimeRange=10  YMin=-1  YMax=0.4000000000000001  SaveName=ScopeData9
  SCOPE_kalmanaltestim : Scope
      settings: TimeRange=13  YMax=1  SaveName=ScopeData25
  Selector4 : Selector  InputPortWidth=3  Indices=[3]
  Selector5 : Selector  InputPortWidth=3  Indices=[3]
  Sum : Sum  Inputs=|++
  WorldToRSinacc : MATLAB Function  TreatAsAtomicUnit=on
  gravity : Constant  Value=[0 0 quad.g]
  invertzaxisGain : Gain  Gain=-1
  outlierBelowFloor : simulink/Logic and Bit Operations/Compare To Constant  relop=>  const=0  OutDataTypeStr=boolean
  prsToAlt_Gain : Gain  Gain=1/quadEDT.altToPrs_Gain
  dz_estimout : Outport
  Z_estimout : Outport  Port=2
  wires:
  att_estimin/1 -> RStoWorldinacc/1(attitude), WorldToRSinacc/1(attitude)
  altSonar_datin/1 -> invertzaxisGain/1
  RStoWorldinacc/1(acc_world) -> Sum/1
  gravity/1 -> Sum/2
  Sum/1 -> Selector5/1
  KalmanFilter_altitude/1 -> Mux1/1, Demux/1
  Mux/1 -> WorldToRSinacc/2(vector)
  Selector5/1 -> KalmanFilter_altitude/1  "ddZ"
  invertzaxisGain/1 -> Mux1/2, KalmanFilter_altitude/2, OutlierHandling/1(altSonarneg_datin)
  Demux/1 -> Bias1/1, Bias/1, Delay2/1, Z_estimout/1  "Z"
  Selector4/1 -> dz_estimout/1  "dz"
  Demux/2 -> Mux/2
  Mux1/1 -> SCOPE_kalmanaltestim/1
  Bias/1 -> Mux1/3
  Bias1/1 -> Mux1/4
  outlierBelowFloor/1 -> KalmanFilter_altitude/4
  prsDelta_datin/1 -> prsToAlt_Gain/1
  prsToAlt_Gain/1 -> SCOPE_altPrs/1, OutlierHandling/2(altPrs_datin)  "altfrompress"
  Delay2/1 -> outlierBelowFloor/1, OutlierHandling/3(Z_estimin)
  OutlierHandling/1(enableKFmeasupdate_flagout) -> KalmanFilter_altitude/3
  dxy_estimtin/1 -> Mux/1
  WorldToRSinacc/1(acc_RS) -> Selector4/1
  Bus Selector2/1 -> Mux2/1  "<ddx>"
  Bus Selector2/2 -> Mux2/2  "<ddy>"
  Bus Selector2/3 -> Mux2/3  "<ddz>"
  sensorIMU_datin/1 -> Bus Selector2/1
  Mux2/1 -> RStoWorldinacc/2(vector)

== system sim_quadrotor/DroneRS_Compensator/Estimator/EstimatorXYPosition ==
  opticalFlow_datin : Inport
  controlModePosVSAtt_flagin : Inport  Port=2
  posVIS_datin : Inport  Port=3
  usePosVIS_flagin : Inport  Port=4
  sensorIMU_datin : Inport  Port=5
  att_estimin : Inport  Port=6
  Z_estimin : Inport  Port=7
  dz_estimin : Inport  Port=8
  EstimatorVelocity : Subsystem
  EstimatorXYPosition : Subsystem
  XY_estimout : Outport
  dxy_estimout : Outport  Port=2
  wires:
  att_estimin/1 -> EstimatorVelocity/4(att_estimin), EstimatorXYPosition/2(att_estimin)
  EstimatorVelocity/1(dxy_estimout) -> EstimatorXYPosition/1(dxy_estimin), dxy_estimout/1
  opticalFlow_datin/1 -> EstimatorVelocity/1(opticalFlow_datin)
  sensorIMU_datin/1 -> EstimatorVelocity/3(sensorIMU_datin)
  Z_estimin/1 -> EstimatorVelocity/2(Z_estimin)
  controlModePosVSAtt_flagin/1 -> EstimatorXYPosition/3(controlModePosVSAtt_flagin)
  dz_estimin/1 -> EstimatorXYPosition/4(dz_estimin)
  posVIS_datin/1 -> EstimatorXYPosition/5(posVIS_datin)
  usePosVIS_flagin/1 -> EstimatorXYPosition/6(usePosVIS_flagin)
  EstimatorXYPosition/1(XY_estimout) -> XY_estimout/1

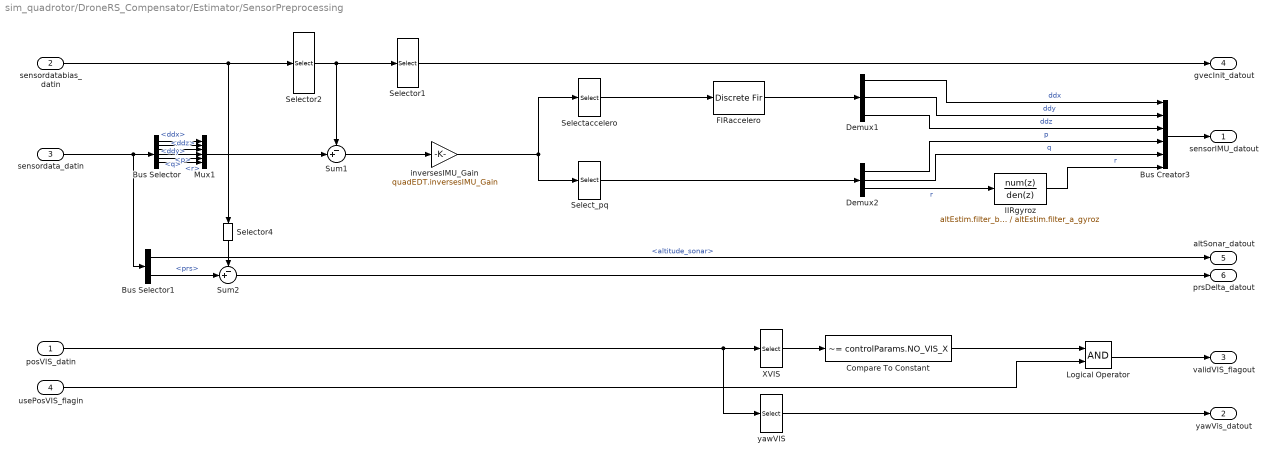
== system sim_quadrotor/DroneRS_Compensator/Estimator/SensorPreprocessing ==
  posVIS_datin : Inport
  sensordatabias_datin : Inport  Port=2
  sensordata_datin : Inport  Port=3
  usePosVIS_flagin : Inport  Port=4
  Bus Creator3 : BusCreator  Inputs=6
  Bus Selector : BusSelector  OutputSignals=ddx,ddy,ddz,p,q,r
  Bus Selector1 : BusSelector  OutputSignals=altitude_sonar,prs
  Compare To Constant : simulink/Logic and Bit Operations/Compare To Constant  relop=~=  const=controlParams.NO_VIS_X  OutDataTypeStr=boolean
  Demux1 : Demux  Outputs=3
  Demux2 : Demux  Outputs=3
  FIRaccelero : DiscreteFir  Coefficients=controlParams.filter_accelero.Coefficients  SampleTime=sampleTime_qcsim
  IIRgyroz : DiscreteFilter  Numerator=altEstim.filter_b_gyroz  Denominator=altEstim.filter_a_gyroz
  Logical Operator : Logic  AllPortsSameDT=off  OutDataTypeStr=boolean
  Mux1 : Mux  Inputs=6
  Select_pq : Selector  InputPortWidth=6  Indices=[4 5 6]
  Selectaccelero : Selector  InputPortWidth=6  Indices=[1 2 3]
  Selector1 : Selector  InputPortWidth=6  Indices=[1:3]
  Selector2 : Selector  InputPortWidth=7  Indices=[1:6]
  Selector4 : Selector  InputPortWidth=7  Indices=[7]
  Sum1 : Sum  Inputs=-+|
  Sum2 : Sum  Inputs=-+|
  XVIS : Selector  InputPortWidth=4
  inversesIMU_Gain : Gain  Gain=quadEDT.inversesIMU_Gain
  yawVIS : Selector  InputPortWidth=4  Indices=4
  sensorIMU_datout : Outport
  yawVis_datout : Outport  Port=2
  validVIS_flagout : Outport  Port=3
  gvecInit_datout : Outport  Port=4
  altSonar_datout : Outport  Port=5
  prsDelta_datout : Outport  Port=6
  wires:
  posVIS_datin/1 -> yawVIS/1, XVIS/1
  Bus Creator3/1 -> sensorIMU_datout/1
  Demux1/1 -> Bus Creator3/1  "ddx"
  Demux1/2 -> Bus Creator3/2  "ddy"
  Demux1/3 -> Bus Creator3/3  "ddz"
  Sum1/1 -> inversesIMU_Gain/1
  Selector2/1 -> Sum1/1, Selector1/1
  Demux2/1 -> Bus Creator3/4  "p"
  Demux2/2 -> Bus Creator3/5  "q"
  inversesIMU_Gain/1 -> Select_pq/1, Selectaccelero/1
  Selectaccelero/1 -> FIRaccelero/1
  FIRaccelero/1 -> Demux1/1
  Demux2/3 -> IIRgyroz/1  "r"
  Selector1/1 -> gvecInit_datout/1
  Select_pq/1 -> Demux2/1
  IIRgyroz/1 -> Bus Creator3/6  "r"
  sensordatabias_datin/1 -> Selector4/1, Selector2/1
  Bus Selector/1 -> Mux1/1  "<ddx>"
  Bus Selector/2 -> Mux1/2  "<ddy>"
  Bus Selector/3 -> Mux1/3  "<ddz>"
  Bus Selector/4 -> Mux1/4  "<p>"
  Bus Selector/5 -> Mux1/5  "<q>"
  Bus Selector/6 -> Mux1/6  "<r>"
  sensordata_datin/1 -> Bus Selector1/1, Bus Selector/1
  Bus Selector1/1 -> altSonar_datout/1  "<altitude_sonar>"
  Selector4/1 -> Sum2/1
  Bus Selector1/2 -> Sum2/2  "<prs>"
  Sum2/1 -> prsDelta_datout/1
  Mux1/1 -> Sum1/2
  XVIS/1 -> Compare To Constant/1
  yawVIS/1 -> yawVis_datout/1
  Logical Operator/1 -> validVIS_flagout/1
  Compare To Constant/1 -> Logical Operator/1
  usePosVIS_flagin/1 -> Logical Operator/2

== system sim_quadrotor/Drone_Sensorsystem/IMU_Pressure/ Noise ==
  statesRTB_datin : Inport
  Add : Sum
  Bus Creator : BusCreator  Inputs='X','Y','Z','yaw','pitch','roll','dx','dy','dz','p','q','r'
  Bus to Vector : BusToVector
  Demux1 : Demux  Outputs=12
  Gaussian Noise Generator : commnoisgen2/Gaussian Noise Generator  m=0  d=quadEDT.noiseStatesSensed_std.^2  s=41  Ts=sampleTime_qcsim  frameBased=off  sampPerFrame=1  orient=off  outDataType=double
  noiseWeights_Gain : Gain  Gain=quadEDT.noiseStatesSensed_weights
  statesRTBnoisy_datout : Outport
  wires:
  Bus Creator/1 -> statesRTBnoisy_datout/1
  Gaussian Noise Generator/1 -> noiseWeights_Gain/1
  Demux1/6 -> Bus Creator/6  "roll"
  Add/1 -> Demux1/1
  Demux1/8 -> Bus Creator/8  "dy"
  Demux1/10 -> Bus Creator/10  "p"
  Demux1/12 -> Bus Creator/12  "r"
  Demux1/2 -> Bus Creator/2  "Y"
  Bus to Vector/1 -> Add/1
  Demux1/3 -> Bus Creator/3  "Z"
  Demux1/7 -> Bus Creator/7  "dx"
  Demux1/9 -> Bus Creator/9  "dz"
  Demux1/4 -> Bus Creator/4  "yaw"
  Demux1/11 -> Bus Creator/11  "q"
  statesRTB_datin/1 -> Bus to Vector/1
  Demux1/5 -> Bus Creator/5  "pitch"
  Demux1/1 -> Bus Creator/1  "X"
  noiseWeights_Gain/1 -> Add/2

== system sim_quadrotor/DroneRS_Compensator/ControllerFSFB/SysteminputConverter/ControlMixerRS ==
  note: NOTE: The controlmixer translates total thrust and the three torque inputs that the controller came up with into 'thrust per motor'.
  T_refin : Inport
  Qyaw_refin : Inport  Port=2
  Qpitch_refin : Inport  Port=3
  Qroll_refin : Inport  Port=4
  Mux2 : Mux
  Product : Product  Multiplication=Matrix(*)  RndMeth=Zero
  Saturation2 : Saturate  UpperLimit=-0.0118  LowerLimit=-0.3235
  TorquetotalThrustToThrustperMotor : Constant  Value=controlParams.Q2Ts
  thrust_refout : Outport
  wires:
  Qroll_refin/1 -> Mux2/4
  Qpitch_refin/1 -> Mux2/3
  Qyaw_refin/1 -> Mux2/2
  T_refin/1 -> Mux2/1
  Product/1 -> Saturation2/1
  TorquetotalThrustToThrustperMotor/1 -> Product/1
  Mux2/1 -> Product/2
  Saturation2/1 -> thrust_refout/1
